simulink library "gbp"  (Simulink 8.1)
settings: Solver=ode45  StartTime=0.0  StopTime=10.0  RelTol=1e-3
undefined symbols (not defined in the file or in its folder): ENUM_GEARPOSN_PN, ENUM_GEARPOSN_R
settings Model: Creator=xsellart  LastModifiedBy=AT015555

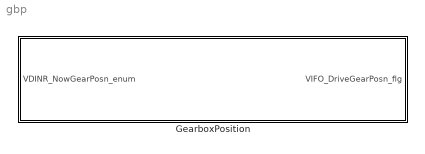
== system gbp ==
  GearboxPosition : Subsystem

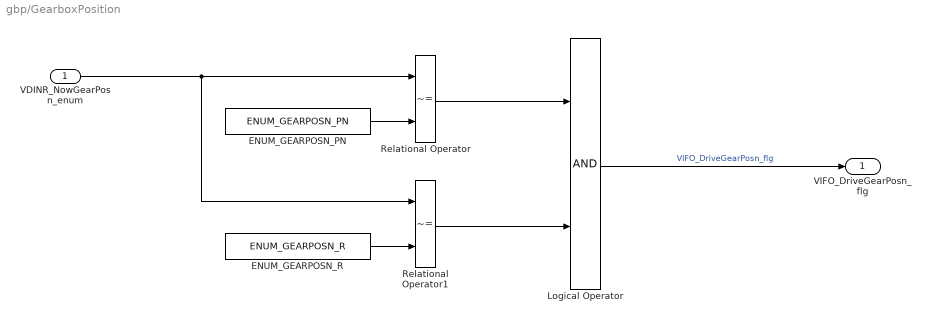
== system gbp/GearboxPosition ==
  VDINR_NowGearPosn_enum : Inport
  ENUM_GEARPOSN_PN : Constant  Value=ENUM_GEARPOSN_PN
  ENUM_GEARPOSN_R : Constant  Value=ENUM_GEARPOSN_R
  Logical Operator : Logic  AllPortsSameDT=off  OutDataTypeStr=boolean
  Relational Operator : RelationalOperator  Operator=~=  OutDataTypeStr=boolean
  Relational Operator1 : RelationalOperator  Operator=~=  OutDataTypeStr=boolean
  VIFO_DriveGearPosn_flg : Outport
  wires:
  VDINR_NowGearPosn_enum/1 -> Relational Operator1/1, Relational Operator/1
  ENUM_GEARPOSN_PN/1 -> Relational Operator/2
  ENUM_GEARPOSN_R/1 -> Relational Operator1/2
  Relational Operator1/1 -> Logical Operator/2
  Relational Operator/1 -> Logical Operator/1
  Logical Operator/1 -> VIFO_DriveGearPosn_flg/1  "VIFO_DriveGearPosn_flg"
